simulink model "y6s"  (R2023b)
settings: Solver=FixedStepAuto  StartTime=0.0  StopTime=50  FixedStep=0.01  RelTol=1e-3
settings Model: Creator=asus  LastModifiedBy=asus

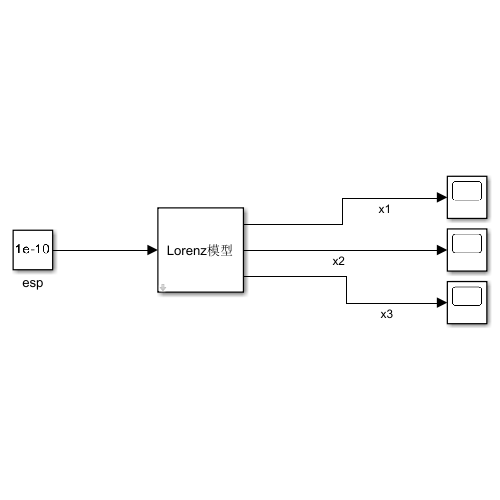
[thumbnail: Simulink's stored preview of the top-level diagram]
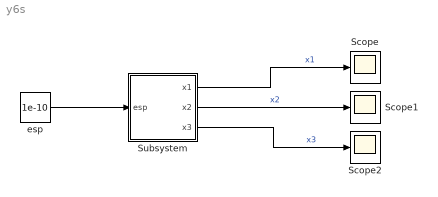
== system y6s ==
  Scope : Scope
  Scope1 : Scope
  Scope2 : Scope
  Subsystem : Subsystem  mask{beta1=8/3, p=10, sei=28, x10=0, x20=0}
      mask prompts: beta1 "beta"; p "rou"; x10 "x1(0)"; x20 "x2(0)"
      mask DialogControl ParameterGroupVar Prompt: 参数
      mask Display: disp('Lorenz模型');
  esp : Constant  Value=1e-10
  wires:
  esp/1 -> Subsystem/1(esp)
  Subsystem/1(x1) -> Scope/1  "x1"
  Subsystem/2(x2) -> Scope1/1  "x2"
  Subsystem/3(x3) -> Scope2/1  "x3"

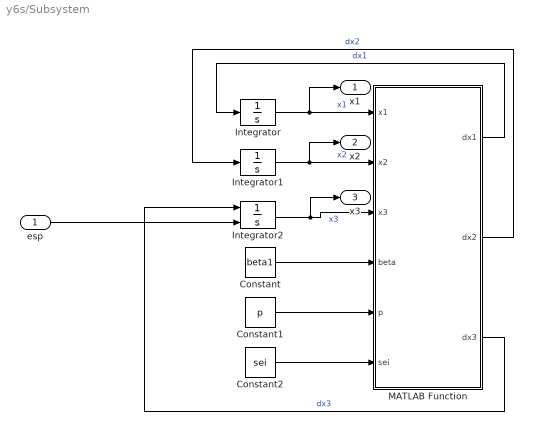
== system y6s/Subsystem ==
  esp : Inport
  Constant : Constant  Value=beta1
  Constant1 : Constant  Value=p
  Constant2 : Constant  Value=sei
  Integrator : Integrator  InitialCondition=x10
  Integrator1 : Integrator  InitialCondition=x20
  Integrator2 : Integrator  InitialConditionSource=external
  MATLAB Function : MATLAB Function  TreatAsAtomicUnit=on
  x1 : Outport
  x2 : Outport  Port=2
  x3 : Outport  Port=3
  wires:
  MATLAB Function/2(dx2) -> Integrator1/1  "dx2"
  Constant2/1 -> MATLAB Function/6(sei)
  Integrator/1 -> x1/1, MATLAB Function/1(x1)  "x1"
  Constant1/1 -> MATLAB Function/5(p)
  Integrator1/1 -> x2/1, MATLAB Function/2(x2)  "x2"
  MATLAB Function/3(dx3) -> Integrator2/1  "dx3"
  MATLAB Function/1(dx1) -> Integrator/1  "dx1"
  Integrator2/1 -> x3/1, MATLAB Function/3(x3)  "x3"
  Constant/1 -> MATLAB Function/4(beta)
  esp/1 -> Integrator2/2

== matlab function y6s/Subsystem/MATLAB Function ==
  data: x1 input; dx1 output; x2 input; x3 input; beta input; p input; sei input; dx2 output; dx3 output
function [dx1,dx2,dx3] = fcn(x1,x2,x3,beta,p,sei)

dx1 = -beta*x1 + x2*x3;
dx2 = -p*x2 + p*x3;
dx3 = -x1*x2 + sei*x2 - x3;
